simulink model "Es1_2slx"  (R2014a)
settings: Solver=ode45  StartTime=0.0  StopTime=30.0  RelTol=1e-3
values from neighbouring files (symbols this model uses):
  Kc = 1    [Es1_2.m]    (also in Es2_1.m; Es2_2.m)
libraries: cstblocks x2
settings Model: Creator=UTENTE  LastModifiedBy=UTENTE

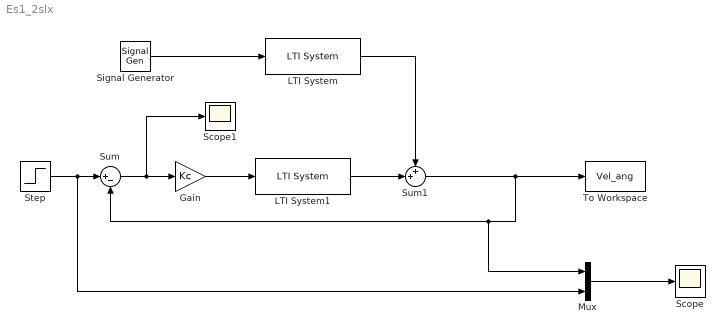
== system Es1_2slx ==
  Gain : Gain  Gain=Kc
  LTI System : cstblocks/LTI System  sys=F2  IC=[]
  LTI System1 : cstblocks/LTI System  sys=F1  IC=[]
  Mux : Mux  Inputs=2
  Scope : Scope
  Scope1 : Scope
  Signal Generator : SignalGenerator  WaveForm=square  Amplitude=0.05  Frequency=0.1
  Step : Step  Time=0  SampleTime=0
  Sum : Sum  Inputs=|+-
  Sum1 : Sum  Inputs=++|
  To Workspace : ToWorkspace  VariableName=Vel_ang  SaveFormat=Timeseries  SampleTime=-1
  wires:
  Signal Generator/1 -> LTI System/1
  LTI System/1 -> Sum1/1
  Sum1/1 -> Mux/1, Sum/2, To Workspace/1
  LTI System1/1 -> Sum1/2
  Gain/1 -> LTI System1/1
  Sum/1 -> Scope1/1, Gain/1
  Mux/1 -> Scope/1
  Step/1 -> Mux/2, Sum/1
